simulink model "ERES_Controller_simulation"  (R2018a)
settings: Solver=VariableStepAuto  StartTime=0.0  StopTime=120  RelTol=1e-3
undefined symbols (not defined in the file): a_lateral_max, atable, atableall, fl_x, fl_y, fr_x, fr_y, high_speed_integrator_saturation_level, high_speed_Ki, high_speed_Kp, num, speed_controller_input_limit, station_error_limit, station_integrator_saturation_level, station_Ki, station_Kp, steer_angle_limited, steer_ratio, t_delay, utable, utableall, Vr, vtable, w1, w2, wheel_base, x0, y0
libraries: simulink x2, Solver_SF x1
settings Model: SimulationMode=rapid-accelerator  Creator=DELL  LastModifiedBy=DELL

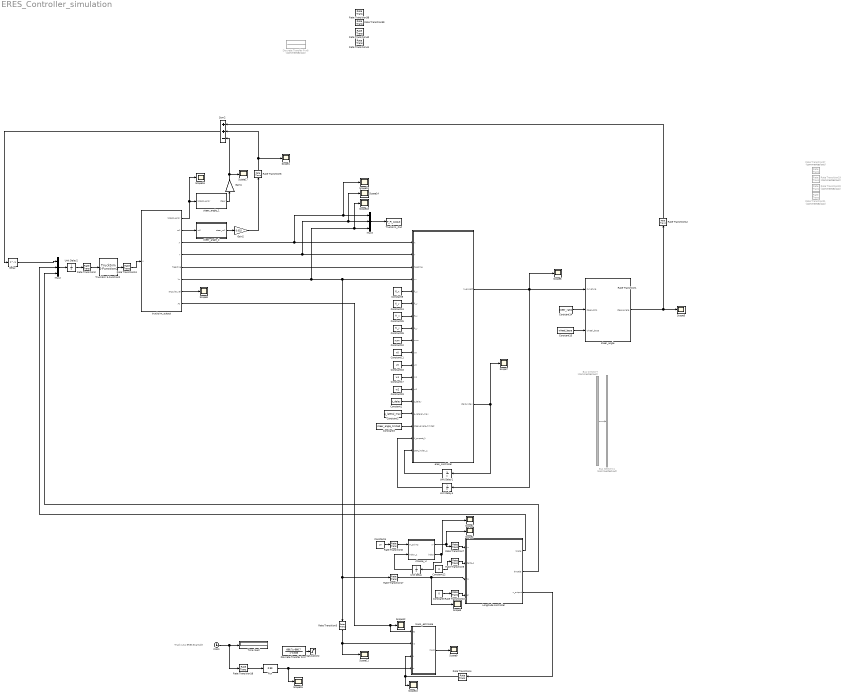
== system ERES_Controller_simulation ==
  note: Truck LKA ERES Example
  Bus Creator3 : BusCreator  Commented=on  Inputs=9
  Bus Selector4 : BusSelector  Commented=on  OutputSignals=num,x0,y0,w1,w2,fl_xe,fl_ye,fr_xe,fr_ye
  Clock : Clock
  Constant1 : Constant  Value=t_delay
  Constant10 : Constant  Value=num
  Constant11 : Constant  Value=x0
  Constant12 : Constant  Value=0
  Constant14 : Constant  Value=steer_ratio
  Constant15 : Constant  Value=wheel_base
  Constant16 : Constant  Value=y0
  Constant17 : Constant  Value=w1
  Constant2 : Constant  Value=a_lateral_max
  Constant23 : Constant  Value=w2
  Constant24 : Constant  Value=fl_y
  Constant25 : Constant  Value=fr_x
  Constant26 : Constant  Value=fr_y
  Constant3 : Constant  Value=steer_angle_limited
  Constant4 : Constant  Value=Vr
  Constant5 : Constant  Value=0
  Constant9 : Constant  Value=fl_x
  Delay : Delay  DelayLength=1  SampleTime=0.01
  Discrete Transfer Fcn7 : DiscreteTransferFcn  Numerator=[666.7 -666.7]  Denominator=[1 -0.333]
  Discrete Transfer Fcn8 : DiscreteTransferFcn  Commented=on  Numerator=[0.004975 0.004975]  Denominator=[1 -0.99]
  Fcn : Fcn  Expr=0.99
  Gain1 : Gain  Gain=0.009
  Gain2 : Gain  Gain=0.015
  Longitude controller : Subsystem
  Mux2 : Mux  Inputs=3
  Mux3 : Mux  Inputs=3
  Rate Transition{1,3..4,6..10,12..13,17..18,38..41} (16 alike) : RateTransition  OutPortSampleTime=0.01
  Rate Transition{19..22} (4 alike) : RateTransition  Commented=on  OutPortSampleTime=0.01
  Rate Transition2 : RateTransition  OutPortSampleTime=0.001
  Saturation2 : Saturate  UpperLimit=1  LowerLimit=-1
  Scope{1..18} (18 alike) : Scope
  Sum2 : Sum  Inputs=++-
  Time (sec) : Display
      settings: Format=bank  Decimation=100
  TruckSim S-Function2 : Solver_SF/TruckSim S-Function2  Priority=1  VehicleCode=s_ss__sss  SIMFILE=simfile.sim
      settings: AttributesFormatString=Vehicle Code: %<VehicleCode>
  Trucksim_Out : ToWorkspace  VariableName=P_PI_output  SampleTime=-1
  Unit Delay : UnitDelay  InitialCondition=1  SampleTime=-1
  Unit Delay1 : UnitDelay  SampleTime=0.01
  Unit Delay2 : UnitDelay  SampleTime=0.01
  Unit Delay4 : UnitDelay  SampleTime=0.01
  choose_vr : MATLAB Function  TreatAsAtomicUnit=on
  eres_controller : MATLAB Function  TreatAsAtomicUnit=on
  mass_estimate : Subsystem
  steer_angle : MATLAB Function  TreatAsAtomicUnit=on
  steer_angle_1 : Subsystem
  steer_angle_2 : Subsystem
  trucksim_output : MATLAB Function  TreatAsAtomicUnit=on
  wires:
  Rate Transition10/1 -> Longitude controller/4(ar)
  Unit Delay/1 -> choose_vr/2(index_1)
  Rate Transition17/1 -> Longitude controller/3(Vx), Scope3/1
  Rate Transition7/1 -> Longitude controller/1(vr)
  Mux2/1 -> Unit Delay2/1
  trucksim_output/6(Vx) -> Scope18/1, Mux3/3, Rate Transition17/1, Rate Transition3/1, eres_controller/4(vx)
  Unit Delay2/1 -> Rate Transition2/1
  Constant15/1 -> steer_angle/3(wheel_base)
  Rate Transition9/1 -> Longitude controller/2(delta_s)
  Rate Transition8/1 -> choose_vr/1(Vr_points)
  Bus Creator3/1 -> Bus Selector4/1
  Constant14/1 -> steer_angle/2(steer_ratio)
  Constant12/1 -> Rate Transition9/1
  Discrete Transfer Fcn7/1 -> Saturation2/1
  trucksim_output/7(angular_vel) -> Scope8/1
  Rate Transition13/1 -> trucksim_output/1(u)
  Constant4/1 -> Rate Transition8/1
  mass_estimate/1(mass) -> Scope9/1
  choose_vr/2(index) -> Unit Delay/1, Scope4/1
  Delay/1 -> Mux2/1
  eres_controller/1(K_expect) -> Scope6/1, steer_angle/1(curvature), Unit Delay4/1
  steer_angle/1(steer_angle) -> Scope5/1, Rate Transition12/1
  Rate Transition18/1 -> Fcn/1
  Longitude controller/2(throttle) -> Mux2/3
  Longitude controller/3(u_output) -> Rate Transition4/1
  Rate Transition3/1 -> Scope11/1, mass_estimate/2(vc)
  Rate Transition4/1 -> mass_estimate/3(u), Scope10/1
  trucksim_output/8(Ac) -> mass_estimate/1(ac), Scope12/1
  Rate Transition2/1 -> TruckSim S-Function2/1
  Constant5/1 -> Rate Transition10/1
  TruckSim S-Function2/1 -> Rate Transition13/1
  Clock/1 -> Rate Transition18/1, Time (sec)/1
  choose_vr/1(vr) -> Scope2/1, Rate Transition7/1
  Fcn/1 -> Scope15/1, mass_estimate/4(w)
  Unit Delay1/1 -> eres_controller/18(start_index_1)
  Constant11/1 -> eres_controller/10(x0)
  Constant16/1 -> eres_controller/11(y0)
  Constant26/1 -> eres_controller/8(fr_y)
  Constant9/1 -> eres_controller/5(fl_x)
  Constant25/1 -> eres_controller/7(fr_x)
  trucksim_output/4(Y) -> Scope14/1, Mux3/2, eres_controller/2(Y)
  Constant17/1 -> eres_controller/12(w1)
  Constant10/1 -> eres_controller/9(num)
  trucksim_output/3(X) -> Scope13/1, Mux3/1, eres_controller/1(X)
  Constant23/1 -> eres_controller/13(w2)
  Constant24/1 -> eres_controller/6(fl_y)
  eres_controller/2(start_index) -> Unit Delay1/1, Scope7/1
  trucksim_output/5(Heading) -> eres_controller/3(heading)
  Constant1/1 -> eres_controller/14(t_delay)
  Constant2/1 -> eres_controller/15(a_lateral_max)
  Constant3/1 -> eres_controller/16(steer_angle_limited)
  Unit Delay4/1 -> eres_controller/17(K_expect_1)
  Mux3/1 -> Trucksim_Out/1
  Gain2/1 -> Rate Transition6/1
  steer_angle_2/1(steer_roll) -> Gain2/1
  trucksim_output/2(roll) -> steer_angle_2/1(roll)
  steer_angle_1/1(steer) -> Gain1/1
  trucksim_output/1(lateral_error) -> Scope16/1, steer_angle_1/1(lateral_error)
  Gain1/1 -> Scope17/1, Sum2/3
  Rate Transition6/1 -> Scope1/1, Sum2/2
  Rate Transition12/1 -> Sum2/1
  Sum2/1 -> Delay/1
  Longitude controller/1(brake) -> Mux2/2

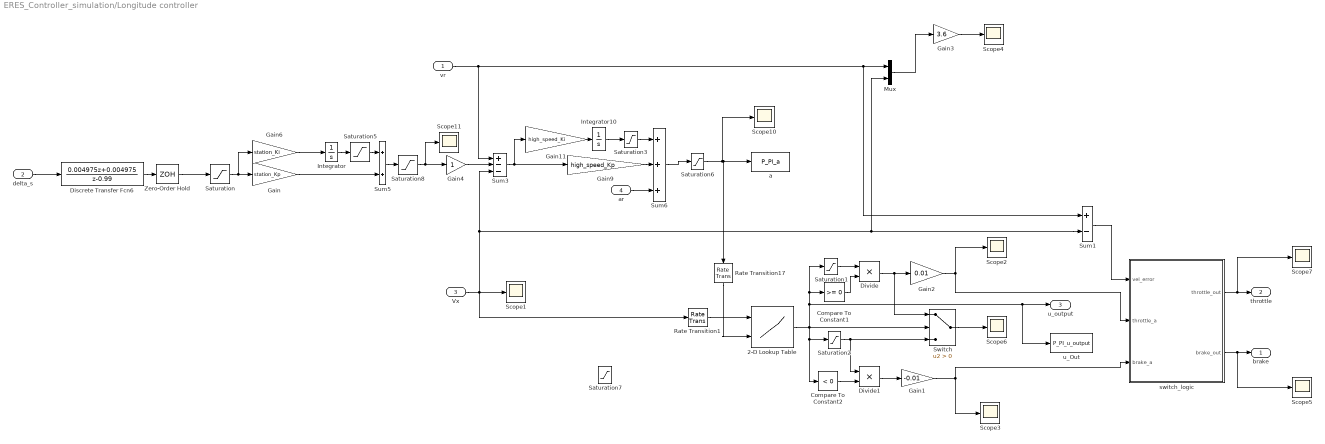
== system ERES_Controller_simulation/Longitude controller ==
  vr : Inport
  delta_s : Inport  Port=2
  Vx : Inport  Port=3
  ar : Inport  Port=4
  2-D Lookup Table : Lookup_n-D  BreakpointsForDimension1=vtable  BreakpointsForDimension2=atable  Table=utableall  ExtrapMethod=Clip  InternalRulePriority=Speed  RndMeth=Simplest  InputSameDT=on
  Compare To Constant1 : simulink/Logic and Bit Operations/Compare To Constant  relop=>=  const=0  OutDataTypeStr=boolean
  Compare To Constant2 : simulink/Logic and Bit Operations/Compare To Constant  relop=<  const=0  OutDataTypeStr=boolean
  Discrete Transfer Fcn6 : DiscreteTransferFcn  Numerator=[0.004975 0.004975]  Denominator=[1 -0.99]
  Divide : Product  Inputs=**
  Divide1 : Product  Inputs=**
  Gain : Gain  Gain=station_Kp
  Gain1 : Gain  Gain=-0.01
  Gain11 : Gain  Gain=high_speed_Ki
  Gain2 : Gain  Gain=0.01
  Gain3 : Gain  Gain=3.6
  Gain4 : Gain
  Gain6 : Gain  Gain=station_Ki
  Gain9 : Gain  Gain=high_speed_Kp
  Integrator : Integrator
  Integrator10 : Integrator
  Mux : Mux  Inputs=2
  Rate Transition1 : RateTransition  OutPortSampleTime=0.01
  Rate Transition17 : RateTransition  OutPortSampleTime=0.01
  Saturation : Saturate  UpperLimit=station_error_limit  LowerLimit=-station_error_limit
  Saturation1 : Saturate  UpperLimit=90  LowerLimit=40*0.2
  Saturation2 : Saturate  UpperLimit=-30*0.2  LowerLimit=-60
  Saturation3 : Saturate  UpperLimit=high_speed_integrator_saturation_level  LowerLimit=-high_speed_integrator_saturation_level
  Saturation5 : Saturate  UpperLimit=station_integrator_saturation_level  LowerLimit=-station_integrator_saturation_level
  Saturation6 : Saturate  UpperLimit=5  LowerLimit=-5
  Saturation7 : Saturate  UpperLimit=100  LowerLimit=0.1
  Saturation8 : Saturate  UpperLimit=speed_controller_input_limit  LowerLimit=-speed_controller_input_limit
  Scope{1..7,10..11} (9 alike) : Scope
  Sum1 : Sum  Inputs=+-
  Sum3 : Sum  Inputs=+--
  Sum5 : Sum
  Sum6 : Sum  Inputs=+++
  Switch : Switch  Criteria=u2 > Threshold
  Zero-Order Hold : ZeroOrderHold  SampleTime=0.01
  a : ToWorkspace  VariableName=P_PI_a  SampleTime=0.01
  switch_logic : Subsystem
  u_Out : ToWorkspace  VariableName=P_PI_u_output  SampleTime=-1
  brake : Outport
  throttle : Outport  Port=2
  u_output : Outport  Port=3
  wires:
  Mux/1 -> Gain3/1
  Saturation3/1 -> Sum6/1
  Gain9/1 -> Sum6/2
  Sum3/1 -> Gain11/1, Gain9/1
  Saturation6/1 -> a/1, Rate Transition17/1, Scope10/1
  Saturation8/1 -> Scope11/1, Gain4/1
  Gain/1 -> Sum5/2
  Integrator10/1 -> Saturation3/1
  vr/1 -> Sum3/1, Sum1/1, Mux/1
  Saturation5/1 -> Sum5/1
  Sum5/1 -> Saturation8/1
  Saturation2/1 -> Divide1/1, Switch/3
  Sum6/1 -> Saturation6/1
  Switch/1 -> Scope6/1
  Gain2/1 -> switch_logic/2(throttle_a), Scope2/1
  Gain1/1 -> switch_logic/3(brake_a), Scope3/1
  2-D Lookup Table/1 -> u_Out/1, u_output/1, Compare To Constant1/1, Saturation1/1, Switch/2, Compare To Constant2/1, Saturation2/1
  Saturation1/1 -> Divide/1
  Compare To Constant1/1 -> Divide/2
  Divide/1 -> Gain2/1, Switch/1
  Compare To Constant2/1 -> Divide1/2
  Divide1/1 -> Gain1/1
  ar/1 -> Sum6/3
  Gain3/1 -> Scope4/1
  Gain11/1 -> Integrator10/1
  Integrator/1 -> Saturation5/1
  Saturation/1 -> Gain6/1, Gain/1
  Gain4/1 -> Sum3/2
  Discrete Transfer Fcn6/1 -> Zero-Order Hold/1
  delta_s/1 -> Discrete Transfer Fcn6/1
  Zero-Order Hold/1 -> Saturation/1
  Vx/1 -> Rate Transition1/1, Sum3/3, Mux/2, Sum1/2, Scope1/1
  Rate Transition17/1 -> 2-D Lookup Table/2
  Rate Transition1/1 -> 2-D Lookup Table/1
  Gain6/1 -> Integrator/1
  Sum1/1 -> switch_logic/1(vel_error)
  switch_logic/2(brake_out) -> Scope5/1, brake/1
  switch_logic/1(throttle_out) -> Scope7/1, throttle/1

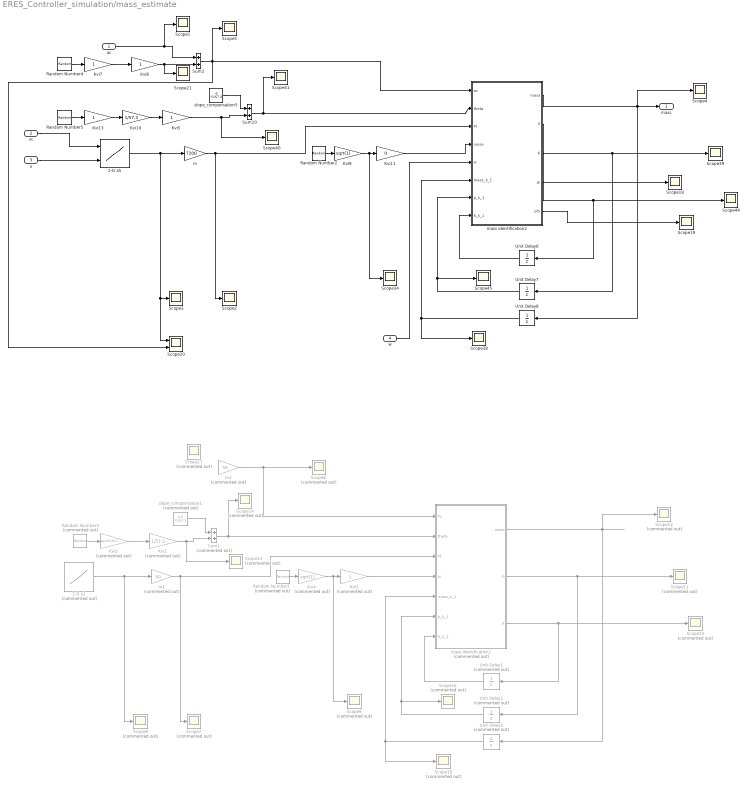
== system ERES_Controller_simulation/mass_estimate ==
  ac : Inport
  vc : Inport  Port=2
  u : Inport  Port=3
  w : Inport  Port=4
  2-D a1 : Lookup_n-D  Commented=on  BreakpointsForDimension1=vtable  BreakpointsForDimension2=utable  BreakpointsForDimension3=[-60 -50]  Table=atableall  InternalRulePriority=Speed  RndMeth=Simplest  InputSameDT=on
  2-D a5 : Lookup_n-D  BreakpointsForDimension1=vtable  BreakpointsForDimension2=utable  BreakpointsForDimension3=[-60 -50]  Table=atableall  InternalRulePriority=Speed  RndMeth=Simplest  InputSameDT=on
  Kvi1 : Gain  Commented=on  Gain=1/57.3
  Kvi10 : Gain  Gain=1/57.3
  Kvi11 : Gain  Gain=0
  Kvi{5,7..8,13} (4 alike) : Gain
  Kvi2 : Gain  Commented=on
  Kvi3 : Gain  Commented=on  Gain=sqrt(0.001)
  Kvi4 : Gain  Commented=on  Gain=sqrt(1)
  Kvi9 : Gain  Gain=sqrt(1)
  Random Number1 : RandomNumber  Commented=on  SampleTime=0.01
  Random Number2 : RandomNumber  Variance=1000000  SampleTime=0.01
  Random Number3 : RandomNumber  Commented=on  Variance=0.1  SampleTime=0.01
  Random Number4 : RandomNumber  Variance=0.001  SampleTime=0.01
  Random Number5 : RandomNumber  SampleTime=0.01
  Scope{1..5,18..19,21,34,38..41,44..45} (15 alike) : Scope
  Scope{6..17} (12 alike) : Scope  Commented=on
  Scope20 : Scope  NumInputPorts=2
  Sum1 : Sum  Commented=on
  Sum10 : Sum
  Sum2 : Sum
  Unit Delay1 : UnitDelay  Commented=on  InitialCondition=1  SampleTime=0.01
  Unit Delay2 : UnitDelay  Commented=on  InitialCondition=100000  SampleTime=0.01
  Unit Delay3 : UnitDelay  Commented=on  InitialCondition=30000  SampleTime=0.01
  Unit Delay6 : UnitDelay  SampleTime=0.01
  Unit Delay7 : UnitDelay  InitialCondition=100000  SampleTime=0.01
  Unit Delay8 : UnitDelay  InitialCondition=25000  SampleTime=0.01
  m : Gain  Gain=7200
  m1 : Gain  Commented=on  Gain=50
  m2 : Gain  Commented=on  Gain=50
  mass identification1 : MATLAB Function  Commented=on  TreatAsAtomicUnit=on  SystemSampleTime=0.01
  mass identification2 : MATLAB Function  TreatAsAtomicUnit=on  SystemSampleTime=0.01
  slope_compensation1 : Constant  Commented=on  Value=0.0 *1/57.3
  slope_compensation5 : Constant  Value=-0 *1/57.3
  mass : Outport
  wires:
  Unit Delay7/1 -> mass identification2/7(p_k_1), Scope45/1
  mass identification2/1(mass) -> Scope4/1, Unit Delay8/1, mass/1
  mass identification2/3(K) -> Unit Delay6/1, Scope44/1
  Unit Delay6/1 -> mass identification2/8(K_k_1)
  Kvi13/1 -> Kvi10/1
  Kvi11/1 -> mass identification2/4(noise)
  Random Number2/1 -> Kvi9/1
  Unit Delay8/1 -> mass identification2/6(mass_k_1), Scope38/1
  slope_compensation5/1 -> Sum10/1
  Kvi10/1 -> Kvi5/1
  Random Number5/1 -> Kvi13/1
  mass identification2/2(P) -> Unit Delay7/1, Scope39/1
  2-D a5/1 -> Scope20/1, Scope3/1, m/1
  vc/1 -> 2-D a5/1
  Kvi9/1 -> Kvi11/1, Scope34/1
  Sum10/1 -> mass identification2/2(theta), Scope41/1
  m/1 -> Scope2/1, mass identification2/3(Ft)
  u/1 -> 2-D a5/2
  m2/1 -> Scope6/1, mass identification1/1(Fc)
  ? -> 2-D a1/2
  m1/1 -> mass identification1/3(Ft), Scope7/1
  Sum1/1 -> Scope14/1, mass identification1/2(theta)
  Kvi4/1 -> Scope9/1, Kvi2/1
  ? -> 2-D a1/1
  2-D a1/1 -> m1/1, Scope8/1
  mass identification1/2(P) -> Scope11/1, Unit Delay2/1
  Random Number3/1 -> Kvi3/1
  Kvi1/1 -> Scope13/1, Sum1/2
  slope_compensation1/1 -> Sum1/1
  Unit Delay3/1 -> Scope10/1, mass identification1/5(mass_k_1)
  Random Number1/1 -> Kvi4/1
  Kvi2/1 -> mass identification1/4(xi)
  ? -> m2/1, Scope17/1
  Kvi3/1 -> Kvi1/1
  Unit Delay1/1 -> mass identification1/7(K_k_1)
  mass identification1/3(K) -> Scope15/1, Unit Delay1/1
  mass identification1/1(mass) -> Unit Delay3/1, Scope12/1
  Unit Delay2/1 -> Scope16/1, mass identification1/6(p_k_1)
  mass identification2/4(gi) -> Scope18/1
  mass identification2/5(phi) -> Scope19/1
  Kvi5/1 -> Sum10/2, Scope40/1
  Random Number4/1 -> Kvi7/1
  Kvi7/1 -> Kvi8/1
  Kvi8/1 -> Scope21/1, Sum2/2
  Sum2/1 -> Scope20/2, Scope5/1, mass identification2/1(ac)
  ac/1 -> Scope1/1, Sum2/1
  w/1 -> mass identification2/5(w)

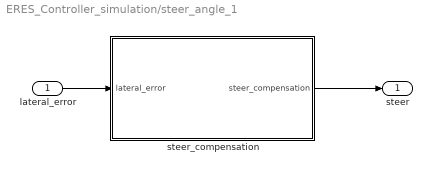
== system ERES_Controller_simulation/steer_angle_1 ==
  lateral_error : Inport
  steer_compensation : MATLAB Function  TreatAsAtomicUnit=on
  steer : Outport
  wires:
  steer_compensation/1(steer_compensation) -> steer/1
  lateral_error/1 -> steer_compensation/1(lateral_error)

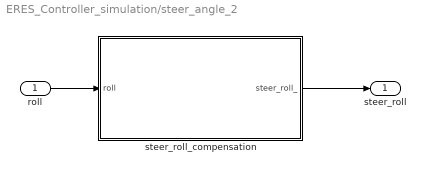
== system ERES_Controller_simulation/steer_angle_2 ==
  roll : Inport
  steer_roll_compensation : MATLAB Function  TreatAsAtomicUnit=on
  steer_roll : Outport
  wires:
  roll/1 -> steer_roll_compensation/1(roll)
  steer_roll_compensation/1(steer_roll_) -> steer_roll/1

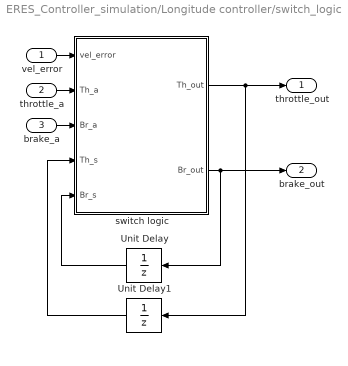
== system ERES_Controller_simulation/Longitude controller/switch_logic ==
  vel_error : Inport
  throttle_a : Inport  Port=2
  brake_a : Inport  Port=3
  Unit Delay : UnitDelay  SampleTime=-1
  Unit Delay1 : UnitDelay  SampleTime=-1
  switch logic : MATLAB Function  TreatAsAtomicUnit=on
  throttle_out : Outport
  brake_out : Outport  Port=2
  wires:
  vel_error/1 -> switch logic/1(vel_error)
  throttle_a/1 -> switch logic/2(Th_a)
  Unit Delay/1 -> switch logic/5(Br_s)
  Unit Delay1/1 -> switch logic/4(Th_s)
  switch logic/1(Th_out) -> Unit Delay1/1, throttle_out/1
  switch logic/2(Br_out) -> Unit Delay/1, brake_out/1
  brake_a/1 -> switch logic/3(Br_a)

== matlab function ERES_Controller_simulation/trucksim_output ==
  data: lateral_error output; roll output; X output; Y output; Heading output; u input; Vx output; angular_vel output; Ac output
function [lateral_error,roll,X,Y,Heading,Vx,angular_vel,Ac]  = fcn(u)

%牵引车信息
X=u(1);
Y=u(2);
Yaw=u(3);
vx=u(4)/3.6;
vy=u(5)/3.6;
Avz=u(6);% unit:deg/s
Heading = Yaw/57.3;  
Vx = vx;%unit:m/s
angular_vel = Avz/57.3;%unit:rad/s
%半挂车信息
X2=u(7);
Y2=u(8);
Yaw2=u(9);
Avz2=u(10);

roll=u(11)/57.3;%unit rad
roll2=u(12);
hitch=u(13);
Ac = u(14) * 9.8;
lateral_error = u(15);

% 车辆坐标系到大地坐标系的转换
% psi1=Yaw/57.3;
% dpsi1=Avz/57.3;
% 
% L=[cos(psi1) -sin(psi1);
%       sin(psi1) cos(psi1)];
% 
% dX=vx*cos(psi1)-vy*sin(psi1);
% dY=vx*sin(psi1)+vy*cos(psi1);%大地系下的速度

== matlab function ERES_Controller_simulation/mass_estimate/mass identification1 ==
  data: mass output; Fc input; theta input; Ft input; xi input; mass_k_1 input; p_k_1 input; K_k_1 input; P output; K output
function [mass,P,K] = fcn(Fc,theta,Ft,xi,mass_k_1,p_k_1,K_k_1)
% Fc = 0;theta = 0;Ft = 0;
na = 1;nb = 1;d = 3; %structure parameters
uk = 0;%initial value of system input
yk = 0;%initial value of system output
L = 1;
g = 9.8;%unit:m/s^2
w = 0.998;
%theta = 0;% slope of the road,unit:degree or rad?

% xi = sqrt(0.1) * randn(L,1);%white noise 
if theta >= 0 
    i = -sin(theta); 
else
    i = sin(theta); 
end
% i = -sin(theta); 
phi = g * i;

Fg = (Fc - Ft - xi) * -1;
% mass = 0;% initial value of the object to be estimated
% persistent mass_last;
% mass_last = 0;
% P = 10^6 * eye(na - 1 + nb - 1 + 1);
% Fg = phi * m + xi; % y(k) = phi(k)' * theta + xi 标准的最小二乘形式
% mass_data 

% RLS algorithm
K = p_k_1 * phi / (w + phi' * p_k_1 * phi);
% mass = mass_last + K * (Fg - phi' * mass_last);
mass = mass_k_1 + K * (Fg - phi' * mass_k_1);
P =1 / w * (eye(na - 1 + nb - 1 + 1) - K * phi') * p_k_1;

% mass_last = mass;

== matlab function ERES_Controller_simulation/mass_estimate/mass identification2 ==
  data: mass output; ac input; theta input; Ft input; noise input; w input; mass_k_1 input; p_k_1 input; K_k_1 input; P output; K output; gi output; phi output
function [mass,P,K,gi,phi] = fcn(ac,theta,Ft,noise,w,mass_k_1,p_k_1,K_k_1)
% Fc = 0;theta = 0;Ft = 0;
na = 1;nb = 1;d = 3; %structure parameters
uk = 0;%initial value of system input
yk = 0;%initial value of system output
L = 1;
g = 9.8;%unit:m/s^2
% w = 0.998;
%theta = 0;% slope of the road,unit:degree or rad?

% xi = sqrt(0.1) * randn(L,1);%white noise 
if theta >= 0 
    i = -sin(theta); 
else
    i = sin(theta); 
end
% i = -sin(theta); 
gi = g*i;
if (ac<0.1) && (ac >0)
    ac = 0.05;
end
if  (ac<0.0) && (ac >-0.1)
         ac = -0.05;
end
phi = g * i +ac;

% Fg = (Fc - Ft - noise) * -1;
Fg =  Ft - noise;
% mass = 0;% initial value of the object to be estimated
% persistent mass_last;
% mass_last = 0;
% P = 10^6 * eye(na - 1 + nb - 1 + 1);
% Fg = phi * m + xi; % y(k) = phi(k-1)' * theta + xi 标准的最小二乘形式
% mass_k_1  = 10000; 

% RLS algorithm
K = p_k_1 * phi / (w + phi' * p_k_1 * phi);
% mass = mass_last + K * (Fg - phi' * mass_last);
mass = mass_k_1 + K * (Fg - phi' * mass_k_1);
P =1 / w * (eye(na - 1 + nb - 1 + 1) - K * phi') * p_k_1;
if mass <=0
    mass = 0;
end

% mass_last = mass;

== matlab function ERES_Controller_simulation/eres_controller ==
  data: X input; Y input; heading input; vx input; K_expect output; fl_x input; fl_y input; fr_x input; fr_y input; num input; x0 input; y0 input; w1 input; w2 input; t_delay input; a_lateral_max input; steer_angle_limited input; K_expect_1 input; start_index output; start_index_1 input
function [K_expect,start_index]  = fcn(X,Y,heading,vx,fl_x,fl_y,fr_x,fr_y,num,x0,y0,w1,w2,t_delay,a_lateral_max,steer_angle_limited,K_expect_1,start_index_1)
%using arc for sampling
% q = floor((klmin - krmax) / delta_k);
p = num;
s = ones(30,1);
s_thresh = 1.2;
klmin = 0.000001;
krmax = 0.000001;
% num = 30;
% fprintf("x_max = %f",x_max);
x_max = 0.00000;
% fprintf("x_max = %f",x_max);
kmax = 1.5;
% klmin = -kmax;
% krmax = kmax;
max_deceleration = 6.0;

C_proximity = ones(num,1);
C_smooth = ones(num,1);
xp_ =  ones(num,1);
sp_ =  ones(num,1);
yp_ =  ones(num,1);
K_expect = 0.0; 
C_p = 0.000001;
C_cost = ones(num,1);
tmp = 0;
index = 1;
%% find the start index 
start_index = 1;
% fprintf("start_index_1 = %f\n",start_index_1);
% start_index = floor(X);

for i = 1:1:length(fl_x)
    if(X < fl_x( i )) || (X< fr_x( i ))
        start_index = i - 1;
        break;
    end
%     break;
end

if start_index <= 1
    start_index = 1;
end

%% convert the coordinates to vehicle coordinate system
fl_x_tmp = zeros(30,1);
fl_y_tmp = zeros(30,1);
fr_x_tmp = zeros(30,1);
fr_y_tmp = zeros(30,1);
for i=1:num
%     fl_xe(i) =fl_x( start_index+i-1 ) ;
    fl_x_tmp(i) = fl_x(start_index + i -1 );
    fl_y_tmp(i) = fl_y(start_index + i -1 );
    fr_x_tmp(i) = fr_x(start_index + i -1 );
    fr_y_tmp(i) = fr_y(start_index + i -1 );
    
end

% left and right line coordinates in global coodinate system
% fl_x_tmp = fl_x( start_index:start_index + num );
% fl_y_tmp = fl_y( start_index:start_index + num );
% fr_x_tmp = fr_x( start_index:start_index + num );
% fr_y_tmp = fr_y( start_index:start_index + num );
% left and right line coordinates in vehicle coodinate system
if X <0
    X = 0;
end
fl_xe = (fl_x_tmp - X) * cos (heading) + (fl_y_tmp - Y) * sin(heading);
fl_ye = (fl_y_tmp - Y) * cos (heading) - (fl_x_tmp - X) * sin(heading);

fr_xe = (fr_x_tmp - X) * cos (heading) + (fr_y_tmp - Y) * sin(heading);
fr_ye = (fr_y_tmp - Y) * cos (heading) - (fr_x_tmp - X) * sin(heading);


%% search control space
% fresh kmax and s_thresh every cycle
% fprintf("vx = %f \n",vx);
% fprintf("a_lateral_max / vx^2 = %f \n",a_lateral_max / vx^2);
% kmax = min((tan(steer_angle_limited/57.3))/4.75 , a_lateral_max / vx^2);
% kmax = min((tan(steer_angle_limited)/57.3)/4.75 , 1.5);
kmax = (tan(steer_angle_limited/57.3))/4.75 ;
% kmax = 1.5;
klmin = kmax;
krmax = -kmax;

% s_thresh = vx ^2 / (2 * max_deceleration) + vx * t_delay;
s_thresh =10;

% fprintf("kmax = %f \n",kmax);
% fprintf("s_thresh = %f \n",s_thresh);

kl = 2 .*  fl_ye ./ (fl_ye.^2 + fl_xe.^2);
kr = 2 .* fr_ye ./ (fr_ye.^2 + fr_xe.^2);

%  the arc length
sl  = 2 .* asin(fl_ye ./ sqrt(fl_xe.^2 + fl_ye.^2)) ./ kl;
sr = 2 .* asin(fr_ye ./ sqrt(fr_xe.^2 + fr_ye.^2)) ./ kr;

for i=1:num 
    s(i)=max(sl(i),sr(i));
%     fprintf("kl (%f) = %f \n",i,kl(i));
%     fprintf("kr (%f) = %f \n",i,kr(i));
%     
%     fprintf("fr_x (%f) = %f \n",i,fr_x(i));
%     fprintf("fr_y (%f) = %f \n",i,fr_y(i));
%     
    
%     if (s(i)<s_thresh)
%         continue;
%     else
%         if (kl(i)<klmin)
%             klmin=kl(i);
% %             fprintf("kl (%f) = %f \n",i,kl(i));
%         end
%         
%         if (kr(i)>-kmax)
%             krmax=kr(i);
%         end
%         
%         x_max=fl_xe(i);%x_max
% %         fprintf("x_max = %f \n",x_max);
%         kr(i)=krmax;
%         kl(i)=klmin;
% %         fprintf("kr (%f) = %f \n",i,kr(i));
%        
%     end
%     %
%     if (kl(i)<kr(i))
%             x_max=fl_xe(i-1);
%         break;
%     else
%         
%     end
%     x_max = 30;



    if kl(i) < kr(i)
        x_max = (i - 1);
        break;
    elseif s(i) < s_thresh
        continue;
    else
        if kl(i) < klmin
            klmin = kl( i );
        end
        
        if kr( i ) > krmax
            krmax = kr( i );
        end
        
        kr( i ) = krmax;
        kl( i ) = klmin;
        x_max = i;
    end
 





end
fprintf("x_max = %f \n",x_max);
%% choose best arc
fprintf("kr(x_max) = %f \n",kr(x_max));
fprintf("kl(x_max) = %f \n",kl(x_max));
% kp = linspace(krmax,klmin,p);
kp = linspace(kr(x_max),kl(x_max),p);
for j = 1:1:(p )
%     fprintf("kp (%f) = %f \n",j,kp(j));
    
    xp_ = linspace(0,x_max,p);
    sp_ = asin(kp(j)*(xp_-x0))/kp(j);
    yp_ = -1/kp(j)*cos(kp(j)*sp_)+1/kp(j)+y0;

    for n = 1:1:length(num)
        tmp = min(abs(yp_( n ) - fl_ye(n)),abs(yp_(n ) - fr_ye(n)));
        C_p = C_p + tmp;
%         fprintf('C_p = %f \n',C_p);
    end

    C_proximity(j) = 1 / C_p;
    C_smooth(j) = (kp(j) - K_expect_1)^2;
    C_p = 0.000001;           
%             plot(xp_,yp_,'y*');%

end

C_cost = w1* C_proximity + w2 * C_smooth;
C_cost_min = C_cost(1);
for m = 1:1:length(C_cost)
    if C_cost(m) <= C_cost_min
        C_cost_min = C_cost(m);
        K_expect = kp(m);
        index = m;
    end 
end

% fprintf('K_expect = %f \n',K_expect);
% fprintf('index = %f \n',index);  


 xy=linspace(0,x_max,100);
 sy=asin(K_expect_1*(xy-x0))/K_expect_1;
 fy=-1/K_expect_1*cos(K_expect_1*sy)+1/K_expect_1+y0;
 plot(xy,fy,'r*')

== matlab function ERES_Controller_simulation/steer_angle_2/steer_roll_compensation ==
  data: roll input; steer_roll_ output
function steer_roll_ = fcn(roll)

steer_roll_ = 9.8 * sin(roll) * 20.34 * 57.3;

== matlab function ERES_Controller_simulation/steer_angle_1/steer_compensation ==
  data: lateral_error input; steer_compensation output
function steer_compensation = fcn(lateral_error)

steer_compensation = 1 * lateral_error * 20.34 * 57.3;

== matlab function ERES_Controller_simulation/steer_angle ==
  data: steer_angle output; curvature input; steer_ratio input; wheel_base input
function steer_angle  = fcn(curvature,steer_ratio,wheel_base)
steer_angle = steer_ratio * atan(wheel_base * curvature) * 180 / pi;

== matlab function ERES_Controller_simulation/choose_vr ==
  data: Vr_points input; vr output; index output; index_1 input
function [vr,index] = fcn(Vr_points,index_1)
index = index_1 + 1;
vr = Vr_points(index + 1);
% fprintf("vr index = %f",index);

== matlab function ERES_Controller_simulation/Longitude controller/switch_logic/switch logic ==
  data: vel_error input; Th_out output; Th_a input; Br_a input; Th_s input; Br_s input; Br_out output
function [Th_out,Br_out] = fcn(vel_error,Th_a,Br_a,Th_s,Br_s)
threshold = 0.01;
Ev = 0.1;
if vel_error < -Ev % deceleration
    if(Th_s > threshold)% throttle control
        Th_out = Th_a;
        Br_out = 0;
    else% brake control
        Th_out = 0;
        Br_out = Br_a;
    end
    
else
    if vel_error > Ev % acceleration
        if(Br_s > threshold) % brake control
            Th_out = 0;
            Br_out = Br_a;
        else % throttle control
            Th_out = Th_a;
            Br_out = 0;
        end
    else % keep region
        if Br_s > threshold
            Th_out = 0;
            Br_out = Br_a;
        else
            if Th_s > threshold
                Th_out = Th_a;
                Br_out = 0; 
            else
                Th_out = 0;
                Br_out = 0;
            end
        end
    end
end
